simulink model "DOF_1"  (R2019b)
settings: Solver=VariableStepAuto  StartTime=0.0  StopTime=10.0  RelTol=1e-3
values from neighbouring files (symbols this model uses):
  c_2 = 7    [DOF_1.mat]    (also in DOF_2.mat)
  k_1 = 2200    [DOF_1.mat]    (also in DOF_2.mat)
  k_2 = 405    [DOF_1.mat]    (also in DOF_2.mat)
  m_1 = 1.5    [DOF_1.mat]    (also in DOF_2.mat)
settings Model: Creator=MASAHIRO  LastModifiedBy=MASAHIRO

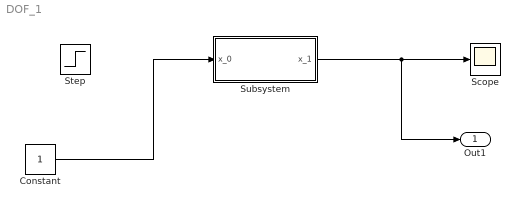
== system DOF_1 ==
  Constant : Constant
  Scope : Scope
  Step : Step  Time=0  After=0.02  SampleTime=0
  Subsystem : Subsystem
  Out1 : Outport
  wires:
  Subsystem/1(x_1) -> Out1/1, Scope/1
  Constant/1 -> Subsystem/1(x_0)

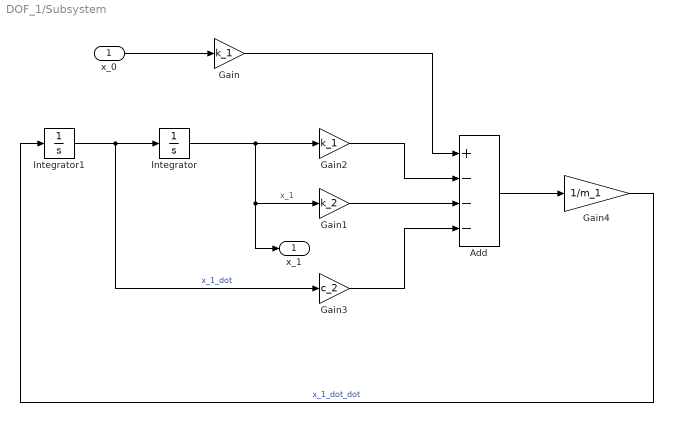
== system DOF_1/Subsystem ==
  x_0 : Inport
  Add : Sum  Inputs=+---
  Gain : Gain  Gain=k_1
  Gain1 : Gain  Gain=k_2
  Gain2 : Gain  Gain=k_1
  Gain3 : Gain  Gain=c_2
  Gain4 : Gain  Gain=1/m_1
  Integrator : Integrator
  Integrator1 : Integrator
  x_1 : Outport
  wires:
  x_0/1 -> Gain/1
  Integrator/1 -> Gain1/1, x_1/1, Gain2/1  "x_1"
  Integrator1/1 -> Gain3/1, Integrator/1  "x_1_dot"
  Gain3/1 -> Add/4
  Gain1/1 -> Add/3
  Gain2/1 -> Add/2
  Gain/1 -> Add/1
  Add/1 -> Gain4/1
  Gain4/1 -> Integrator1/1  "x_1_dot_dot"
